simulink model "Practica3"  (R2020b)
settings: Solver=VariableStepAuto  StartTime=0.0  StopTime=10.0  RelTol=1e-3
model workspace (MAT data in the model file):
  Kr = 100
  Kt = 0.5
  Kv = 0.5
  L1 = 1
  L2 = 0.6
  Ra = 0.3
  fv1 = 2.5
  fv2 = 1.5
  m1 = 10
  m2 = 4
settings Model: Creator=Danie  LastModifiedBy=Danie

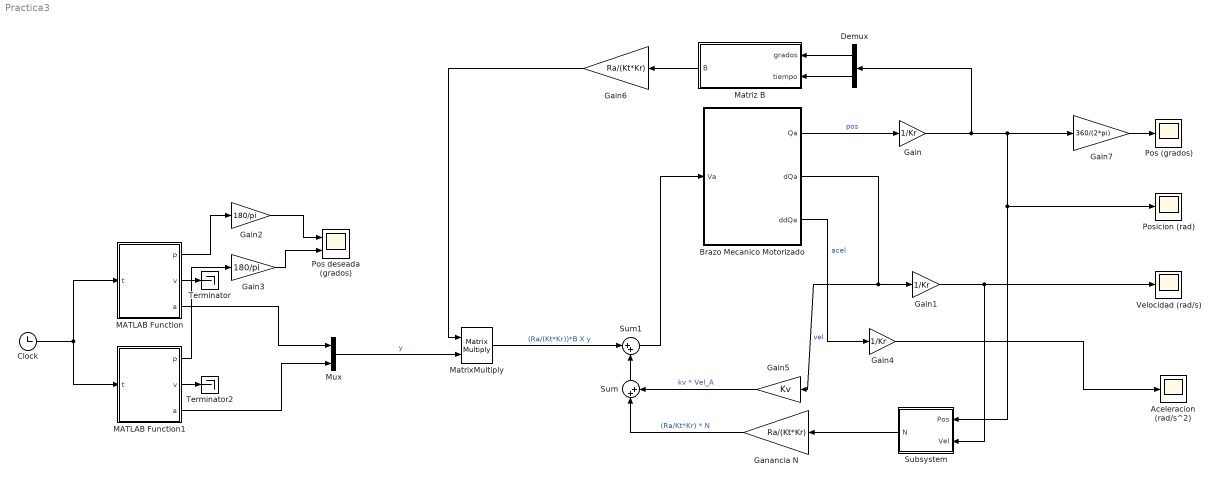
== system Practica3 ==
  Aceleracion (rad/s^2) : Scope
  Brazo Mecanico Motorizado : Subsystem  mask{Ra=0.3, kt=0.5, kv=0.5, Kr1=100, Kr2=100, sat_rpm=1500}
      mask prompts: Ra "Resistencia de la armadura del motor (Ra)"; kt "Constante de conversiòn de tensiòn-par (kt)"; kv "Constante de la fuerzaq contra-electromotriz (kv)"; Kr1 "Reductor del actuador 1 (Kr1)"; Kr2 "Reductor del actuador 2 (Kr2)"; sat_rpm "rpm max actuadores"
  Clock : Clock
  Demux : Demux  Outputs=2
  Gain : Gain  Gain=1/Kr
  Gain1 : Gain  Gain=1/Kr
  Gain2 : Gain  Gain=180/pi
  Gain3 : Gain  Gain=180/pi
  Gain4 : Gain  Gain=1/Kr
  Gain5 : Gain  Gain=Kv
  Gain6 : Gain  Gain=Ra/(Kt*Kr)
  Gain7 : Gain  Gain=360/(2*pi)
  "Ganancia N " : Gain  Gain=Ra/(Kt*Kr)
  MATLAB Function : MATLAB Function  TreatAsAtomicUnit=on  mask{theta0=0, thetaf=10, tf=4}
      mask prompts: theta0 "Pos Inicial (grados)"; thetaf "Pos final (grados)"; tf "Tiempo Final"
  MATLAB Function1 : MATLAB Function  TreatAsAtomicUnit=on  mask{theta0=0, thetaf=5, tf=4}
      mask prompts: theta0 "Pos Inicial (grados)"; thetaf "Pos final (grados)"; tf "Tiempo Final"
  MatrixMultiply : Product  Multiplication=Matrix(*)
  Matriz B : MATLAB Function  TreatAsAtomicUnit=on
  Mux : Mux  Inputs=2
  Pos (grados) : Scope
  Pos deseada (grados) : Scope  NumInputPorts=2
  Posicion (rad) : Scope
  Subsystem : Subsystem
  Sum : Sum  Inputs=|++
  Sum1 : Sum  Inputs=|++
  Terminator : Terminator
  Terminator2 : Terminator
  "Velocidad (rad/s) " : Scope
  wires:
  MATLAB Function/3(a) -> Mux/1
  Clock/1 -> MATLAB Function/1(t), MATLAB Function1/1(t)
  MATLAB Function/2(v) -> Terminator/1
  MATLAB Function1/1(p) -> Gain3/1
  MATLAB Function/1(p) -> Gain2/1
  Gain3/1 -> Pos deseada (grados)/2
  Gain2/1 -> Pos deseada (grados)/1
  Gain7/1 -> Pos (grados)/1
  "Ganancia N "/1 -> Sum/1  "(Ra/Kt*Kr) * N"
  Brazo Mecanico Motorizado/1(Qa) -> Gain/1  "pos"
  Subsystem/1("N ") -> "Ganancia N "/1
  Demux/2 -> Matriz B/2(tiempo)
  Matriz B/1(B) -> Gain6/1
  MATLAB Function1/3(a) -> Mux/2
  Brazo Mecanico Motorizado/2(dQa) -> Gain5/1, Gain1/1  "vel"
  Demux/1 -> Matriz B/1(grados)
  Gain/1 -> Demux/1, Gain7/1, Subsystem/1(Pos), Posicion (rad)/1
  Mux/1 -> MatrixMultiply/2  "y"
  Gain4/1 -> Aceleracion (rad/s^2)/1
  Sum/1 -> Sum1/2
  Brazo Mecanico Motorizado/3(ddQa) -> Gain4/1  "acel"
  MATLAB Function1/2(v) -> Terminator2/1
  Sum1/1 -> Brazo Mecanico Motorizado/1(Va)
  Gain5/1 -> Sum/2  "kv * Vel_A"
  Gain1/1 -> Subsystem/2(Vel), "Velocidad (rad/s) "/1
  Gain6/1 -> MatrixMultiply/1
  MatrixMultiply/1 -> Sum1/1  "(Ra/(Kt*Kr))*B X y"

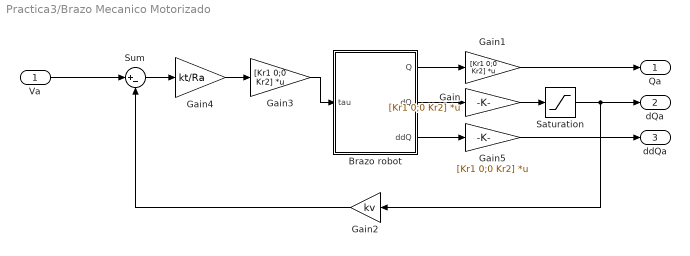
== system Practica3/Brazo Mecanico Motorizado ==
  Va : Inport
  Brazo robot : Subsystem  mask{m1=10, m2=4, L1=1, L2=0.6, fv1=2.5, fv2=1.5}
      mask prompts: m1 "Masa 1"; m2 "Masa 2"; L1 "Longitud 1"; L2 "Longitud 2"; fv1 "Friccion 1"; fv2 "Friccion 2"
  Gain{,1,3,5} (4 alike) : Gain  Gain=[Kr1 0;0 Kr2]  Multiplication=Matrix(K*u) (u vector)
  Gain2 : Gain  Gain=kv
  Gain4 : Gain  Gain=kt/Ra
  Saturation : Saturate  UpperLimit=sat_rpm*2*pi/60  LowerLimit=-sat_rpm*2*pi/60
  Sum : Sum  Inputs=|+-
  Qa : Outport
  dQa : Outport  Port=2
  ddQa : Outport  Port=3
  wires:
  Brazo robot/1(Q) -> Gain1/1
  Brazo robot/2(dQ) -> Gain/1
  Gain/1 -> Saturation/1
  Gain2/1 -> Sum/2
  Sum/1 -> Gain4/1
  Gain4/1 -> Gain3/1
  Gain3/1 -> Brazo robot/1(tau)
  Gain1/1 -> Qa/1
  Va/1 -> Sum/1
  Saturation/1 -> Gain2/1, dQa/1
  Brazo robot/3(ddQ) -> Gain5/1
  Gain5/1 -> ddQa/1

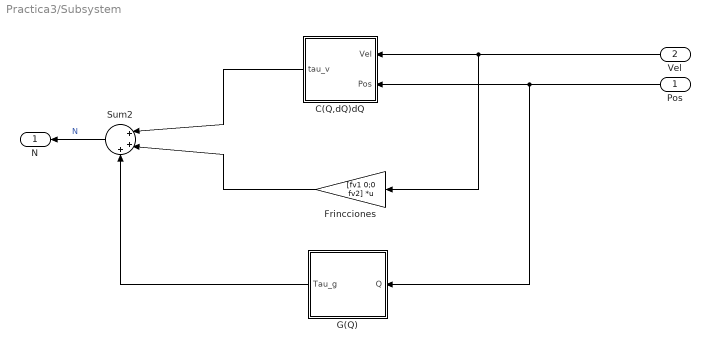
== system Practica3/Subsystem ==
  Pos : Inport
  Vel : Inport  Port=2
  C(Q,dQ)dQ : Subsystem
  Frincciones : Gain  Gain=[fv1 0;0 fv2]  Multiplication=Matrix(K*u)  SaturateOnIntegerOverflow=on  OutDataTypeStr=Inherit: Same as input  ParamDataTypeStr=Inherit: Same as input
  G(Q) : Subsystem
  Sum2 : Sum  Inputs=|+++
  "N " : Outport
  wires:
  Frincciones/1 -> Sum2/2
  G(Q)/1(Tau_g) -> Sum2/3
  Vel/1 -> C(Q,dQ)dQ/1(Vel), Frincciones/1
  C(Q,dQ)dQ/1(tau_v) -> Sum2/1
  Sum2/1 -> "N "/1  "N"
  Pos/1 -> G(Q)/1(Q), C(Q,dQ)dQ/2("Pos ")

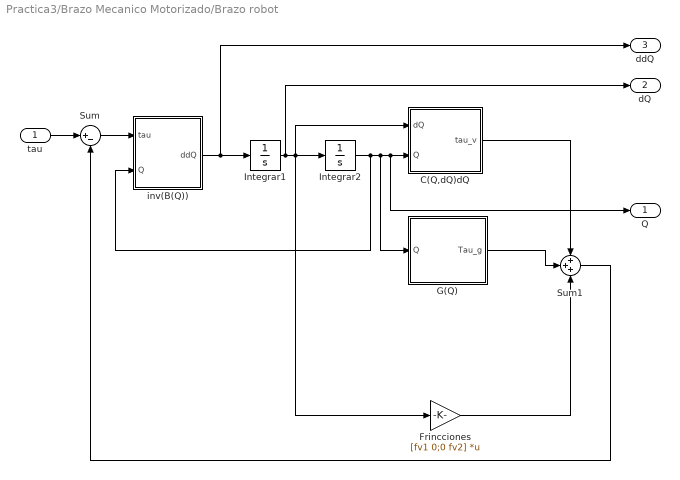
== system Practica3/Brazo Mecanico Motorizado/Brazo robot ==
  tau : Inport
  C(Q,dQ)dQ : Subsystem
  Frincciones : Gain  Gain=[fv1 0;0 fv2]  Multiplication=Matrix(K*u)  SaturateOnIntegerOverflow=on  OutDataTypeStr=Inherit: Same as input  ParamDataTypeStr=Inherit: Same as input
  G(Q) : Subsystem
  Integrar1 : Integrator  InitialCondition=[0,0]
  Integrar2 : Integrator  InitialCondition=[0 0]
  Sum : Sum  Inputs=|+-  SaturateOnIntegerOverflow=on
  Sum1 : Sum  Inputs=+++  SaturateOnIntegerOverflow=on
  inv(B(Q)) : Subsystem
  Q : Outport
  dQ : Outport  Port=2
  ddQ : Outport  Port=3
  wires:
  tau/1 -> Sum/1
  Sum/1 -> inv(B(Q))/1(tau)
  inv(B(Q))/1(ddQ) -> Integrar1/1, ddQ/1
  Integrar1/1 -> Integrar2/1, C(Q,dQ)dQ/1(dQ), Frincciones/1, dQ/1
  Integrar2/1 -> C(Q,dQ)dQ/2(Q), Q/1, G(Q)/1(Q), inv(B(Q))/2(Q)
  C(Q,dQ)dQ/1(tau_v) -> Sum1/1
  G(Q)/1(Tau_g) -> Sum1/2
  Sum1/1 -> Sum/2
  Frincciones/1 -> Sum1/3

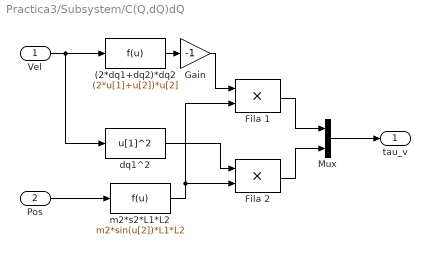
== system Practica3/Subsystem/C(Q,dQ)dQ ==
  Vel : Inport
  "Pos " : Inport  Port=2
  (2*dq1+dq2)*dq2 : Fcn  Expr=(2*u[1]+u[2])*u[2]
  Fila 1 : Product  SaturateOnIntegerOverflow=on  OutDataTypeStr=Inherit: Same as first input
  Fila 2 : Product  SaturateOnIntegerOverflow=on  OutDataTypeStr=Inherit: Same as first input
  Gain : Gain  Gain=-1  SaturateOnIntegerOverflow=on  OutDataTypeStr=Inherit: Same as input  ParamDataTypeStr=Inherit: Same as input
  Mux : Mux  Inputs=2
  dq1^2 : Fcn  Expr=u[1]^2
  m2*s2*L1*L2 : Fcn  Expr=m2*sin(u[2])*L1*L2
  tau_v : Outport
  wires:
  "Pos "/1 -> m2*s2*L1*L2/1
  m2*s2*L1*L2/1 -> Fila 2/2, Fila 1/2
  Vel/1 -> (2*dq1+dq2)*dq2/1, dq1^2/1
  dq1^2/1 -> Fila 2/1
  Fila 1/1 -> Mux/1
  Fila 2/1 -> Mux/2
  Mux/1 -> tau_v/1
  (2*dq1+dq2)*dq2/1 -> Gain/1
  Gain/1 -> Fila 1/1

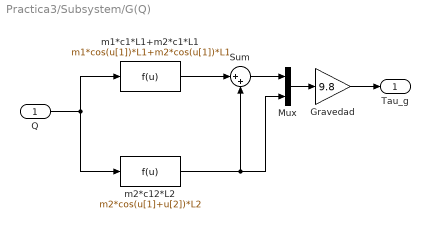
== system Practica3/Subsystem/G(Q) ==
  Q : Inport
  Gravedad : Gain  Gain=9.8  SaturateOnIntegerOverflow=on  OutDataTypeStr=Inherit: Same as input  ParamDataTypeStr=Inherit: Same as input
  Mux : Mux  Inputs=2
  Sum : Sum  Inputs=|++  SaturateOnIntegerOverflow=on
  m1*c1*L1+m2*c1*L1 : Fcn  Expr=m1*cos(u[1])*L1+m2*cos(u[1])*L1
  m2*c12*L2 : Fcn  Expr=m2*cos(u[1]+u[2])*L2
  Tau_g : Outport
  wires:
  m1*c1*L1+m2*c1*L1/1 -> Sum/1
  m2*c12*L2/1 -> Sum/2, Mux/2
  Sum/1 -> Mux/1
  Q/1 -> m1*c1*L1+m2*c1*L1/1, m2*c12*L2/1
  Gravedad/1 -> Tau_g/1
  Mux/1 -> Gravedad/1

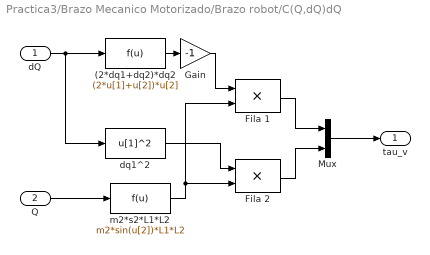
== system Practica3/Brazo Mecanico Motorizado/Brazo robot/C(Q,dQ)dQ ==
  dQ : Inport
  Q : Inport  Port=2
  (2*dq1+dq2)*dq2 : Fcn  Expr=(2*u[1]+u[2])*u[2]
  Fila 1 : Product  SaturateOnIntegerOverflow=on  OutDataTypeStr=Inherit: Same as first input
  Fila 2 : Product  SaturateOnIntegerOverflow=on  OutDataTypeStr=Inherit: Same as first input
  Gain : Gain  Gain=-1  SaturateOnIntegerOverflow=on  OutDataTypeStr=Inherit: Same as input  ParamDataTypeStr=Inherit: Same as input
  Mux : Mux  Inputs=2
  dq1^2 : Fcn  Expr=u[1]^2
  m2*s2*L1*L2 : Fcn  Expr=m2*sin(u[2])*L1*L2
  tau_v : Outport
  wires:
  Q/1 -> m2*s2*L1*L2/1
  m2*s2*L1*L2/1 -> Fila 2/2, Fila 1/2
  dQ/1 -> (2*dq1+dq2)*dq2/1, dq1^2/1
  dq1^2/1 -> Fila 2/1
  Fila 1/1 -> Mux/1
  Fila 2/1 -> Mux/2
  Mux/1 -> tau_v/1
  (2*dq1+dq2)*dq2/1 -> Gain/1
  Gain/1 -> Fila 1/1

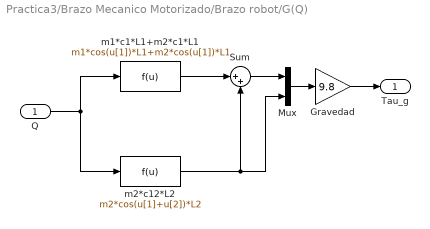
== system Practica3/Brazo Mecanico Motorizado/Brazo robot/G(Q) ==
  Q : Inport
  Gravedad : Gain  Gain=9.8  SaturateOnIntegerOverflow=on  OutDataTypeStr=Inherit: Same as input  ParamDataTypeStr=Inherit: Same as input
  Mux : Mux  Inputs=2
  Sum : Sum  Inputs=|++  SaturateOnIntegerOverflow=on
  m1*c1*L1+m2*c1*L1 : Fcn  Expr=m1*cos(u[1])*L1+m2*cos(u[1])*L1
  m2*c12*L2 : Fcn  Expr=m2*cos(u[1]+u[2])*L2
  Tau_g : Outport
  wires:
  m1*c1*L1+m2*c1*L1/1 -> Sum/1
  m2*c12*L2/1 -> Sum/2, Mux/2
  Sum/1 -> Mux/1
  Q/1 -> m1*c1*L1+m2*c1*L1/1, m2*c12*L2/1
  Gravedad/1 -> Tau_g/1
  Mux/1 -> Gravedad/1

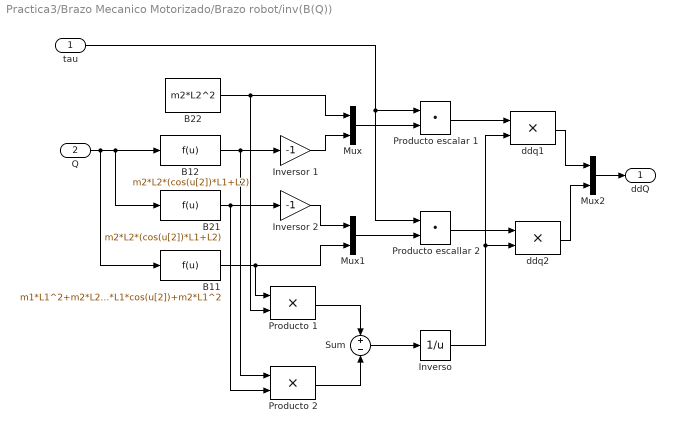
== system Practica3/Brazo Mecanico Motorizado/Brazo robot/inv(B(Q)) ==
  tau : Inport
  Q : Inport  Port=2
  B11 : Fcn  Expr=m1*L1^2+m2*L2^2+2*m2*L2*L1*cos(u[2])+m2*L1^2
  B12 : Fcn  Expr=m2*L2*(cos(u[2])*L1+L2)
  B21 : Fcn  Expr=m2*L2*(cos(u[2])*L1+L2)
  B22 : Constant  Value=m2*L2^2
  Inverso : Math  Operator=reciprocal  SignedPower=on  SaturateOnIntegerOverflow=on
  Inversor 1 : Gain  Gain=-1  SaturateOnIntegerOverflow=on  OutDataTypeStr=Inherit: Same as input  ParamDataTypeStr=Inherit: Same as input
  Inversor 2 : Gain  Gain=-1  SaturateOnIntegerOverflow=on  OutDataTypeStr=Inherit: Same as input  ParamDataTypeStr=Inherit: Same as input
  Mux : Mux  Inputs=2
  Mux1 : Mux  Inputs=2
  Mux2 : Mux  Inputs=2
  Producto 1 : Product  SaturateOnIntegerOverflow=on  OutDataTypeStr=Inherit: Same as first input
  Producto 2 : Product  SaturateOnIntegerOverflow=on  OutDataTypeStr=Inherit: Same as first input
  Producto escalar 1 : DotProduct  InputSameDT=on  OutDataTypeStr=Inherit: Inherit via internal rule
  Producto escallar 2 : DotProduct  InputSameDT=on  OutDataTypeStr=Inherit: Inherit via internal rule
  Sum : Sum  Inputs=+-  SaturateOnIntegerOverflow=on
  ddq1 : Product  SaturateOnIntegerOverflow=on  OutDataTypeStr=Inherit: Same as first input
  ddq2 : Product  SaturateOnIntegerOverflow=on  OutDataTypeStr=Inherit: Same as first input
  ddQ : Outport
  wires:
  Q/1 -> B12/1, B21/1, B11/1
  B12/1 -> Inversor 1/1, Producto 2/1
  B21/1 -> Inversor 2/1, Producto 2/2
  B22/1 -> Mux/1, Producto 1/2
  Inversor 1/1 -> Mux/2
  Inversor 2/1 -> Mux1/1
  B11/1 -> Mux1/2, Producto 1/1
  Mux/1 -> Producto escalar 1/2
  tau/1 -> Producto escalar 1/1, Producto escallar 2/1
  Mux1/1 -> Producto escallar 2/2
  Producto 1/1 -> Sum/1
  Producto 2/1 -> Sum/2
  Sum/1 -> Inverso/1
  Producto escalar 1/1 -> ddq1/1
  Producto escallar 2/1 -> ddq2/1
  Inverso/1 -> ddq1/2, ddq2/2
  ddq1/1 -> Mux2/1
  ddq2/1 -> Mux2/2
  Mux2/1 -> ddQ/1

== matlab function Practica3/MATLAB Function ==
  data: theta0 parameter; p output; thetaf parameter; tf parameter; t input; v output; a output
%%Tema 5 Ejercicio 1
% Calcular y dibujar la trayectoria definida por un polinomio cúbico
% Con velocidad inicial y final 0
function [p,v,a]  = pol3 (theta0,thetaf,tf,t)
    thetaff = thetaf*(2*pi)/360;
    %Parámetros resultantes de resolver las ecuaciones
    a0= theta0;
    a1= 0;
    a2= (3/tf.^2)*(thetaff-theta0);
    a3= -(2/tf.^3)*(thetaff-theta0);
    %% Ecuaciones de posicion, velocidad y aceleracion
    p= a0+a1*t+a2*t^2+a3*t^3;
    v= a1+2*a2.*t+3*a3*t.^2;
    a= 2*a2+6*a3.*t;
       
    %subplot(3,1,1), plot(p,t); title('Posición'); ylabel('º');
    %subplot(3,1,2), plot(v,t); title('Velocidad');ylabel('º/s');
    %subplot(3,1,3), plot(a,t); title('Aceleración');ylabel('º/s^2');

== matlab function Practica3/Matriz B ==
  data: grados input; B output; tiempo input
function B = MatrizB(grados,tiempo)

m1 =10;
m2 = 4;
L1 = 1;
L2 = 0.6;
fr1 = 2.5;
fr2 = 1.5;


B11 = m1*L1^2 + m2*L2^2 + 2*m2*L2*L1*cos(tiempo) + m2*L1^2; 
B12 = m2*L2*(cos(tiempo)*L1+L2);
B21 = m2*L2*(cos(tiempo)*L1+L2);
B22 = m2*L2^2;

B = [B11, B12; B21, B22];

== matlab function Practica3/MATLAB Function1 ==
  data: theta0 parameter; p output; thetaf parameter; tf parameter; t input; v output; a output
%%Tema 5 Ejercicio 1
% Calcular y dibujar la trayectoria definida por un polinomio cúbico
% Con velocidad inicial y final 0
function [p,v,a]  = pol3 (theta0,thetaf,tf,t)
    thetaff = thetaf*(2*pi)/360;
    %Parámetros resultantes de resolver las ecuaciones
    a0= theta0;
    a1= 0;
    a2= (3/tf.^2)*(thetaff-theta0);
    a3= -(2/tf.^3)*(thetaff-theta0);
    %% Ecuaciones de posicion, velocidad y aceleracion
    p= a0+a1*t+a2*t^2+a3*t^3;
    v= a1+2*a2.*t+3*a3*t.^2;
    a= 2*a2+6*a3.*t;
       
    %subplot(3,1,1), plot(p,t); title('Posición'); ylabel('º');
    %subplot(3,1,2), plot(v,t); title('Velocidad');ylabel('º/s');
    %subplot(3,1,3), plot(a,t); title('Aceleración');ylabel('º/s^2');
